simulink model "BuckConverterLoad"  (R2016a)
settings: Solver=ode14x  StartTime=0.0  StopTime=0.1  RelTol=1e-3
libraries: fl_lib x18, nesl_utility x10, elec_lib x1
settings Model: Creator=enes_  LastModifiedBy=enes_

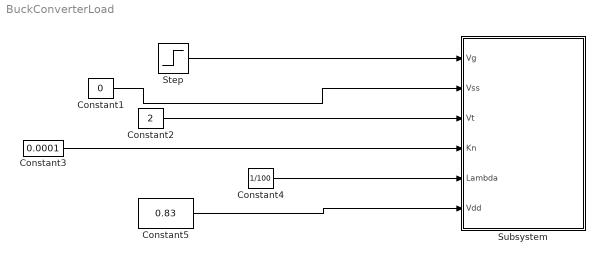
== system BuckConverterLoad ==
  Constant1 : Constant  Value=0
  Constant2 : Constant  Value=2
  Constant3 : Constant  Value=0.0001
  Constant4 : Constant  Value=1/100
  Constant5 : Constant  Value=0.83
  Step : Step  Time=0.01  After=6
  Subsystem : Subsystem
  wires:
  Step/1 -> Subsystem/1(Vg)
  Constant1/1 -> Subsystem/2(Vss)
  Constant2/1 -> Subsystem/3(Vt)
  Constant3/1 -> Subsystem/4(Kn)
  Constant4/1 -> Subsystem/5(Lambda)
  Constant5/1 -> Subsystem/6(Vdd)

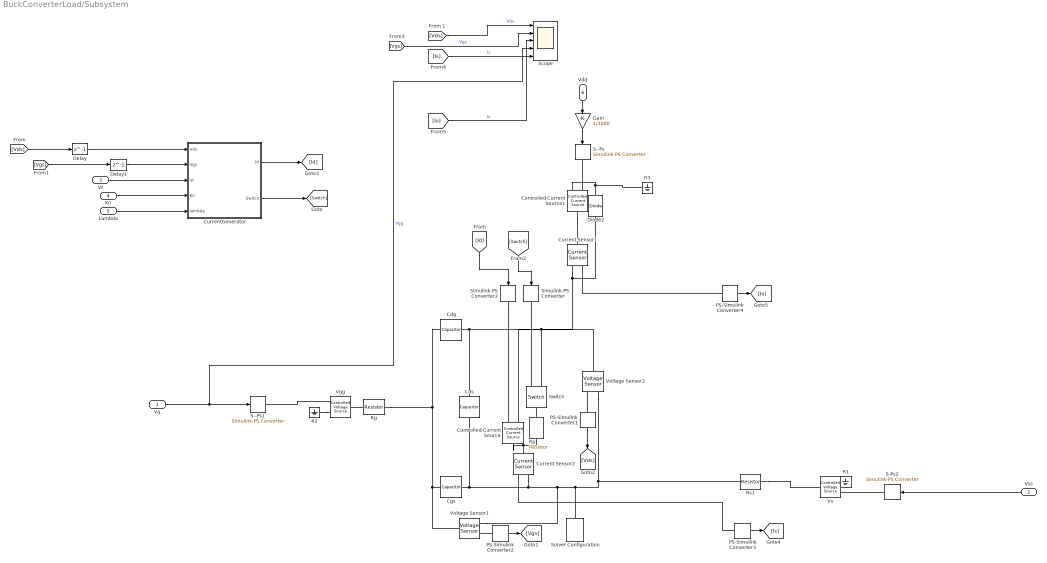
== system BuckConverterLoad/Subsystem ==
  Vg : Inport
  Vss : Inport  Port=2
  Vt : Inport  Port=3
  Kn : Inport  Port=4
  Lambda : Inport  Port=5
  Vdd : Inport  Port=6
  Cdg : fl_lib/Electrical/Electrical Elements/Capacitor  c=130 pF  r=1e-6 Ohm  g=0 1/Ohm  i_specify=off  i_priority=None  i=0 A  v_specify=off  v_priority=None  v=0 V  vc_specify=off  vc_priority=High  vc=0 V
  Cds : fl_lib/Electrical/Electrical Elements/Capacitor  c=100 pF  r=1e-6 Ohm  g=0 1/Ohm  i_specify=off  i_priority=None  i=0 A  v_specify=off  v_priority=None  v=0 V  vc_specify=off  vc_priority=High  vc=0 V
  Cgs : fl_lib/Electrical/Electrical Elements/Capacitor  c=1400 pF  r=1e-6 Ohm  g=0 1/Ohm  i_specify=off  i_priority=None  i=0 A  v_specify=off  v_priority=None  v=0 V  vc_specify=off  vc_priority=High  vc=0 V
  Controlled Current Source : fl_lib/Electrical/Electrical Sources/Controlled Current Source
  Controlled Current Source1 : fl_lib/Electrical/Electrical Sources/Controlled Current Source
  Current Sensor1 : fl_lib/Electrical/Electrical Sensors/Current Sensor
  Current Sensor2 : fl_lib/Electrical/Electrical Sensors/Current Sensor
  CurrentGenerator : MATLAB Function  TreatAsAtomicUnit=on
  Delay : Delay  DelayLength=1  InitialCondition=0  UseCircularBuffer=on
  Delay1 : Delay  DelayLength=1  InitialCondition=0  UseCircularBuffer=on
  Diode2 : elec_lib/Semiconductor Devices/Diode  ModelType=1  Vf=0.6 V  Ron=0.3 Ohm  Goff=1e-8 S  Rz=0.3 Ohm  Vz=50 V  C_PWL=5 pF  prmExp=1  I12=[ 0.0137 0.545 ] A  V12=[ 0.6 0.7 ] V  I1=0.0137 A  V1=0.6 V  RS=0.01 Ohm  IS=1e-12 A  Tmeas=25 degC  ec=1  BV=Inf V  C_param=1  CJ0=5 pF  VJ=1 V  Mgrad=0.5  Vvec=[ 0.1 10 100 ] V  Cvec=[ 3.5 1 0.4 ] pF  FC=0.5  Q_param=1  Irrm=-7.15 A  iF=4 A  didt=-750 A/us  trr=115 ns  TT=50 ns  tau=100 ns  T_param=1  IS_T2=1.25e-7 A  I1_T2=0.245 A  V1_T2=0.5 V  Tmeas2=125 degC  EG_param=1  EG=1.11 eV  XTI_param=1  XTI=3  dBVdT=0 V/K  Tdevice=25 degC  Rth=[ 0 10 ] K/W  thermal_mass_parameterization=1  thermal_mass=[ 0 1 ] J/K  thermal_time_constant=[ 0 10 ] s  thermal_mass_initial_temperatures=[ 25 25 ] degC
  Gain : Gain  Gain=1/1000
  PS-Simulink Converter{1..4} (4 alike) : nesl_utility/PS-Simulink Converter  PhysicalDomain=network_engine_domain  SubClassName=ps_output  LeftPortType=input  RightPortType=output  PseudoPeriodic=off  Frequencies=[]  Unit=1  AffineConversion=off
  R1 : fl_lib/Electrical/Electrical Elements/Electrical Reference
  R2 : fl_lib/Electrical/Electrical Elements/Electrical Reference
  R3 : fl_lib/Electrical/Electrical Elements/Electrical Reference
  Rg : fl_lib/Electrical/Electrical Elements/Resistor  R=200 kOhm  i_specify=off  i_priority=None  i=0 A  v_specify=off  v_priority=None  v=0 V
  Rp : fl_lib/Electrical/Electrical Elements/Resistor  R=10 Ohm  i_specify=off  i_priority=None  i=0 A  v_specify=off  v_priority=None  v=0 V
  Rs1 : fl_lib/Electrical/Electrical Elements/Resistor  R=2 kOhm  i_specify=off  i_priority=None  i=0 A  v_specify=off  v_priority=None  v=0 V
  S--Ps : nesl_utility/Simulink-PS Converter  PhysicalDomain=network_engine_domain  SubClassName=ps_input  LeftPortType=input  RightPortType=output  PseudoPeriodic=off  Frequencies=[]  NoiseDistribution=none  NoiseParameters=[]  Unit=1  AffineConversion=off  InputFiltering=off  SimscapeFilterOrder=1  InputFilterTimeConstant=0.001  UdotUserProvided=1
  S--Ps1 : nesl_utility/Simulink-PS Converter  PhysicalDomain=network_engine_domain  SubClassName=ps_input  LeftPortType=input  RightPortType=output  PseudoPeriodic=off  Frequencies=[]  NoiseDistribution=none  NoiseParameters=[]  Unit=1  AffineConversion=off  InputFiltering=off  SimscapeFilterOrder=1  InputFilterTimeConstant=0.001  UdotUserProvided=1
  S-Ps2 : nesl_utility/Simulink-PS Converter  PhysicalDomain=network_engine_domain  SubClassName=ps_input  LeftPortType=input  RightPortType=output  PseudoPeriodic=off  Frequencies=[]  NoiseDistribution=none  NoiseParameters=[]  Unit=1  AffineConversion=off  InputFiltering=off  SimscapeFilterOrder=1  InputFilterTimeConstant=0.001  UdotUserProvided=1
  Scope : Scope  NumInputPorts=5
  Simulink-PS Converter : nesl_utility/Simulink-PS Converter  PhysicalDomain=network_engine_domain  SubClassName=ps_input  LeftPortType=input  RightPortType=output  PseudoPeriodic=off  Frequencies=[]  NoiseDistribution=none  NoiseParameters=[]  Unit=1  AffineConversion=off  InputFiltering=off  SimscapeFilterOrder=1  InputFilterTimeConstant=0.001  UdotUserProvided=1
  Simulink-PS Converter2 : nesl_utility/Simulink-PS Converter  PhysicalDomain=network_engine_domain  SubClassName=ps_input  LeftPortType=input  RightPortType=output  PseudoPeriodic=off  Frequencies=[]  NoiseDistribution=none  NoiseParameters=[]  Unit=1  AffineConversion=off  InputFiltering=off  SimscapeFilterOrder=1  InputFilterTimeConstant=0.001  UdotUserProvided=1
  Solver Configuration : nesl_utility/Solver Configuration  PhysicalDomain=network_engine_domain  SubClassName=solver  LeftPortType=input  RightPortType=generic  Accelerate=off  Tones=[]  Harmonics=[]  SimulateNoise=off  Profile=off  UseLocalSampling=off  EnableSwitchedLinearOptims=on  FrequencyDomain=off  UseCCode=off  RelTol=0.001  AbsTol=1e-06  MinStep=1e-09  ToWorkspace=off  RevertToSquareIcSolve=off  NumHomotopyIterations=100  PhasorMode=off  PhasorModeNumHarmonics=1  OverrideAbsTol=off  DoDC=off  ResidualTolerance=1e-09  UseLocalSolver=off  LocalSolverChoice=NE_BACKWARD_EULER_ADVANCER  LocalSolverSampleTime=0.001  DoFixedCost=off  MaxNonlinIter=3  MaxModeIter=2  LinearAlgebra=Sparse  DelaysMemoryBudget=1024  AutomaticFiltering=on  FilteringTimeConstant=0.001
  Switch : fl_lib/Electrical/Electrical Elements/Switch  R_closed=0.01 Ohm  G_open=1e-8 1/Ohm  Threshold=0.5  i_specify=off  i_priority=None  i=0 A  v_specify=off  v_priority=None  v=0 V
  Vgg : fl_lib/Electrical/Electrical Sources/Controlled Voltage Source
  Voltage Sensor1 : fl_lib/Electrical/Electrical Sensors/Voltage Sensor
  Voltage Sensor2 : fl_lib/Electrical/Electrical Sensors/Voltage Sensor
  Vs : fl_lib/Electrical/Electrical Sources/Controlled Voltage Source
  wires:
  Vt/1 -> CurrentGenerator/3(Vt)
  [Vds] -> Delay/1
  Lambda/1 -> CurrentGenerator/5(lambda)
  Vdd/1 -> Gain/1
  [Id] -> Simulink-PS Converter2/1
  Kn/1 -> CurrentGenerator/4(Kn)
  [Switch] -> Simulink-PS Converter/1
  CurrentGenerator/2(Switch) -> [Switch]
  Vg/1 -> Scope/4, S--Ps1/1  "Vgg"
  PS-Simulink Converter2/1 -> [Vgs]
  [Is] -> Scope/3  "Is"
  [Vgs] -> Scope/2  "Vgs"
  CurrentGenerator/1(Id) -> [Id]
  [Vds] -> Scope/1  "Vds"
  PS-Simulink Converter1/1 -> [Vds]
  Vss/1 -> S-Ps2/1
  [Vgs] -> Delay1/1
  Delay/1 -> CurrentGenerator/1(Vds)
  Delay1/1 -> CurrentGenerator/2(Vgs)
  Gain/1 -> S--Ps/1
  PS-Simulink Converter3/1 -> [Is]
  PS-Simulink Converter4/1 -> [Io]
  [Io] -> Scope/5  "Io"
  connections:
  PS-Simulink Converter2/LConn1 -- Voltage Sensor1/RConn1
  PS-Simulink Converter1/LConn1 -- Voltage Sensor2/RConn1
  Rp/LConn1 -- Switch/LConn1
  Simulink-PS Converter/RConn1 -- Switch/RConn1
  Vgg/RConn1 -- S--Ps1/RConn1
  Simulink-PS Converter2/RConn1 -- Controlled Current Source/RConn1
  Rg/RConn1 -- Voltage Sensor1/LConn1 -- Cgs/LConn1 -- Cdg/RConn1
  R1/LConn1 -- Vs/RConn2
  S-Ps2/RConn1 -- Vs/RConn1
  Rg/LConn1 -- Vgg/LConn1
  R2/LConn1 -- Vgg/RConn2
  Diode2/RConn1 -- R3/LConn1 -- Controlled Current Source1/RConn2
  Controlled Current Source1/RConn1 -- S--Ps/RConn1
  PS-Simulink Converter3/LConn1 -- Current Sensor2/RConn1
  Controlled Current Source1/LConn1 -- Current Sensor1/LConn1
  PS-Simulink Converter4/LConn1 -- Current Sensor1/RConn1
  Switch/RConn2 -- Controlled Current Source/RConn2 -- Current Sensor1/RConn2 -- Diode2/LConn1
  Voltage Sensor2/LConn1 -- Cds/LConn1 -- Cdg/LConn1
  Rs1/RConn1 -- Vs/LConn1
  Cds/RConn1 -- Cgs/RConn1 -- Current Sensor2/RConn2 -- Voltage Sensor2/RConn2 -- Rs1/LConn1 -- Solver Configuration/RConn1 -- Voltage Sensor1/RConn2
  Controlled Current Source/LConn1 -- Current Sensor2/LConn1 -- Rp/RConn1

== matlab function BuckConverterLoad/Subsystem/CurrentGenerator ==
  data: Vds input; Id output; Vgs input; Vt input; Kn input; lambda input; Switch output
function [Id,Switch] = fcn(Vds,Vgs,Vt,Kn,lambda)
%#codegen
% Vds: Drain-to-source voltage in V
% Vgs: Gate-to-source voltage in V
% Vt: Threshold Voltage in V
% Kn: Devices parameter in A/V^2
% Lambda: Early voltage in V^-1

% Id: Drain-to-Source Current
% Switch : determines the on-off state of switch
Current=0;
SwitchStat=0;
GSVt= Vgs-Vt; % it determines transistor on or off

OnStat=Vds-Vgs+Vt; % it determines transistor is sat or linear

if GSVt>0
    
    if OnStat>0
        % SaturationRegion
       Current = 0.5*Kn*(GSVt^2)*(1+lambda*Vds);
       SwitchStat= 0;
    else
        % Triode region
        %Current=Kn*((GSVt*Vds)-(0.5*Vds*Vds))*(1+lambda*Vds);
        SwitchStat=1;
        Current=0;        
    end
    
    
    
    
else
    % cut-off region
    Current=0;
    SwitchStat=0;
    
end

Id=Current;
Switch=SwitchStat;
